simulink model "P_3_step_error"  (R2021a)
settings: Solver=VariableStepAuto  StartTime=0.0  StopTime=25  RelTol=1e-3
settings Model: Creator=alamg  LastModifiedBy=alamg

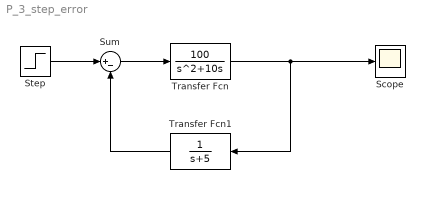
== system P_3_step_error ==
  Scope : Scope
  Step : Step  SampleTime=0
  Sum : Sum  Inputs=|+-
  Transfer Fcn : TransferFcn  Numerator=[100]  Denominator=[1 10 0]
  Transfer Fcn1 : TransferFcn  Denominator=[1 5]
  wires:
  Transfer Fcn/1 -> Transfer Fcn1/1, Scope/1
  Transfer Fcn1/1 -> Sum/2
  Sum/1 -> Transfer Fcn/1
  Step/1 -> Sum/1
